simulink model "controller"  (R2012b)
settings: Solver=FixedStepDiscrete  StartTime=0.0  StopTime=inf  RelTol=1e-3
InitFcn:
  | initRov14;
values from neighbouring files (symbols this model uses):
  k = [ 20   5   15 ... (first row only)    [initRov14.m]    (also in initSharedMem.m = [ 0*20   0*5   0*15)
undefined symbols (not defined in the file or in its folder): DiscIntNeverNeededParam, m, qDes
libraries: WBCLibrary x10, utility x1
settings Model: Creator=daniele  LastModifiedBy=daniele

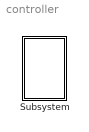
== system controller ==
  Subsystem : Subsystem  mask{robotName='icubGazeboSim', Ts=0.01, localName='dynamicBalancing'}
      mask prompts: robotName "robot name"; localName "module name"

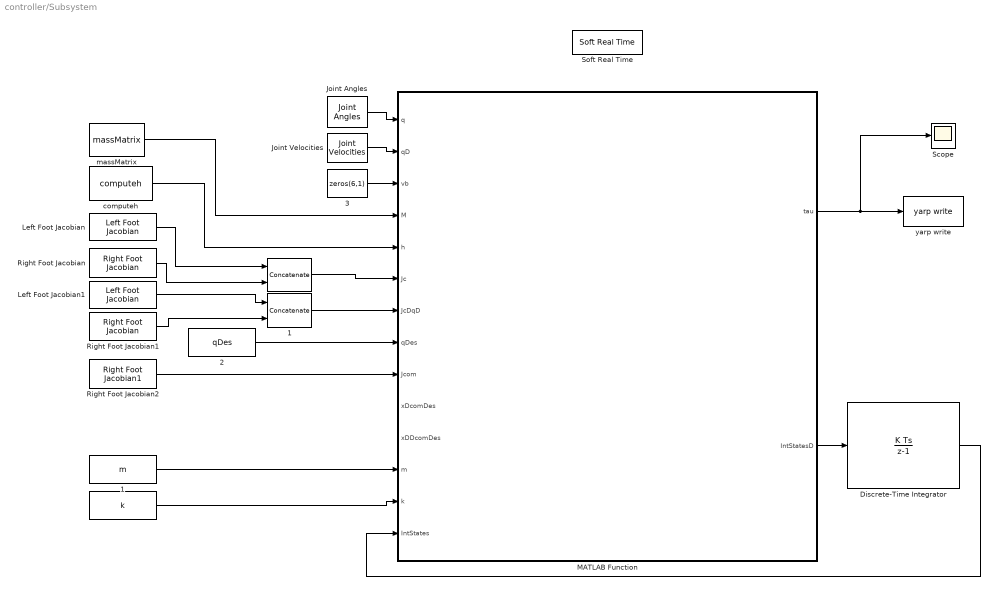
== system controller/Subsystem ==
  " " : Constant  Value=k
  " 2" : Constant  Value=qDes
  " 3" : Constant  Value=zeros(6,1)
  " " : Concatenate  Mode=Multidimensional array
  "  1" : Constant  Value=m
  " 1" : Concatenate  Mode=Multidimensional array
  Discrete-Time Integrator : DiscreteIntegrator  SampleTime=-1  ICPrevOutput=DiscIntNeverNeededParam  ICPrevScaledInput=DiscIntNeverNeededParam
  Joint Angles : WBCLibrary/wholeBodyStates/Joint Angles  robotName=robotName  localName=localName
  Joint Velocities : WBCLibrary/wholeBodyStates/Joint Velocities  robotName=robotName  localName=localName
  Left Foot Jacobian : WBCLibrary/wholeBodyModel/Jacobians/Left Foot Jacobian  robotName=robotName  localName=localName
  Left Foot Jacobian1 : WBCLibrary/wholeBodyModel/Jacobians/Left Foot Jacobian  robotName=robotName  localName=localName
  MATLAB Function : MATLAB Function  TreatAsAtomicUnit=on
  Right Foot Jacobian : WBCLibrary/wholeBodyModel/Jacobians/Right Foot Jacobian  robotName=robotName  localName=localName
  Right Foot Jacobian1 : WBCLibrary/wholeBodyModel/Jacobians/Right Foot Jacobian  robotName=robotName  localName=localName
  Right Foot Jacobian2 : WBCLibrary/wholeBodyModel/Jacobians/Right Foot Jacobian1  robotName=robotName  localName=localName
  Scope : Scope
  Soft Real Time : utility/Soft Real Time  x=Ts
  computeh : WBCLibrary/wholeBodyModel/Dynamics/computeh  val=7  robotname=robotName  localname='simulink'
  massMatrix : WBCLibrary/wholeBodyModel/Dynamics/massMatrix  val=8  robotname=robotName  localname='simulink'
  yarp write : WBCLibrary/Utilities/yarp write  port_name='/test:o'
  wires:
  Joint Velocities/1 -> MATLAB Function/2(qD)
  computeh/1 -> MATLAB Function/5(h)
  massMatrix/1 -> MATLAB Function/4(M)
  Right Foot Jacobian1/1 -> " 1"/2
  " 2"/1 -> MATLAB Function/8(qDes)
  MATLAB Function/1(tau) -> Scope/1, yarp write/1
  Joint Angles/1 -> MATLAB Function/1(q)
  Right Foot Jacobian2/1 -> MATLAB Function/9(Jcom)
  " 3"/1 -> MATLAB Function/3(vb)
  " "/1 -> MATLAB Function/6(Jc)
  " "/1 -> MATLAB Function/13(k)
  "  1"/1 -> MATLAB Function/12(m)
  MATLAB Function/2(IntStatesD) -> Discrete-Time Integrator/1
  Discrete-Time Integrator/1 -> MATLAB Function/14(IntStates)
  Left Foot Jacobian/1 -> " "/1
  Right Foot Jacobian/1 -> " "/2
  " 1"/1 -> MATLAB Function/7(JcDqD)
  Left Foot Jacobian1/1 -> " 1"/1

== matlab function controller/Subsystem/MATLAB Function ==
  data: q input; qD input; vb input; M input; h input; Jc input; JcDqD input; tau output; qDes input; Jcom input; xDcomDes input; xDDcomDes input; m input; k input; IntStates input; IntStatesD output
function [tau,IntStatesD] = fcn(q, qD, vb, M, h, Jc, JcDqD, qDes, Jcom, xDcomDes, xDDcomDes, m, k, IntStates)
%#codegen

PINV_TOL = 1e-5;
g        = 9.81;

n     =  size(M,1);
Mb    =  M(1:6,1:6);
MbInv = inv(Mb);
Mbj   = M(1:6,7:end); 
Mj    = M(7:end,7:end);
U     = [eye(6) , zeros(6,n)];
Jcb   = Jc*U';
SBar  = [  -MbInv*Mbj 
           eye(n)      ];
NjInv = Mj - Mbj'*MbInv*Mb;

% Gravity affects only linear motions of the CoM
grav = [0;0;m*g;zeros(3,1)];

JcSBar     = Jc*SBar;
JcSBarPinv = pinv(JcSBar, PINV_TOL);

% Definition of reference accelerations for CoM and Joints that ensure
% stabilization of desired trajectories xDcomDes and qDes 
xDcom   = Jcom*[vb;qD];
nu_star = xDDcomDes - k(1,1)*(xDcom - xDcomDes) - k(1,2)*IntStates(n+1:end);
q_star  =        - k(2,1)*qD           - k(2,2)*(q - qDes) - k(2,3)*IntStates(1:n) ;

% Updates for integral terms
IntStatesD = [(q - qDes);(xDcom - xDcomDes)];

A     = [eye(6) eye(6)];
Apinv = 0.5*A';
NA    = 0.5*[eye(6),-eye(6);-eye(6),eye(6)];


% The following expressions for Ic and IcD hold only if the control 
% objective is the stabilization of the CoM's position
Ic  = [ m*eye(3),zeros(3)
       zeros(3),zeros(3)];
IcD = zeros(6);

FeedCoM             = grav + IcD*xDcom + Ic*nu_star;
% EquaLeftRifghFoot   = -0.5*[eye(3),zeros(3),-eye(3),zeros(3);zeros(3,12);-eye(3),zeros(3),eye(3),zeros(3);zeros(3,12)]*Apinv*FeedCoM;  
EquaLeftRifghFoot   = zeros(size(A,2),1);
fd                  = Apinv*FeedCoM + NA*EquaLeftRifghFoot;

fd(4:6)    = zeros(3,1); 
fd(10:end) = zeros(3,1);

LambdaStar = JcSBarPinv*(Jcb*MbInv*(h(1:6) - Jcb'*fd) - JcDqD);

NPi = eye(n) - JcSBarPinv*JcSBar;

LambdaStar = LambdaStar + NPi * q_star;

tau = NjInv*LambdaStar + SBar'*h - (JcSBar)'*fd;
